simulink model "Connor"  (R2022b)
settings: Solver=VariableStepAuto  StartTime=0.0  StopTime=1  MaxStep=0.0001  RelTol=1e-3
values from neighbouring files (symbols this model uses):
  batteryTempCurve = (1 - batteryCoef *      (batteryTempX / maxBatteryTemp) .^ 2)    [red_crayon.m]
  batteryTempX = 0 : maxBatteryTemp / STEP_SIZE : maxBatteryTemp    [red_crayon.m]
  motorTempCurve = 150 -  (motorTempX - minMotorTemp) .^ 2 .* (150) / (maxMotorTemp - minMotorTemp)^2    [red_crayon.m]
  motorTempX = minMotorTemp : (maxMotorTemp-minMotorTemp) / STEP_SIZE : maxMotorTemp    [red_crayon.m]
undefined symbols (not defined in the file or in its folder): CENTER_STEER_ANGLE_MAX, deadband_angle, theta_left, theta_right, theta_sweep
libraries: dspstat3 x1
settings Model: Creator=Inver  LastModifiedBy=dagge
settings ModelReferenceCC: EnableRefExpFcnMdlSchedulingChecks=on

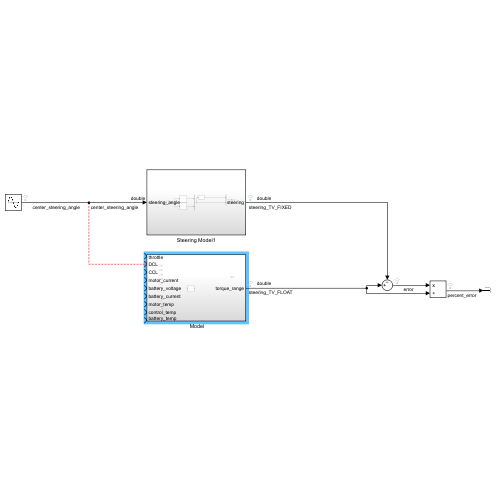
[thumbnail: Simulink's stored preview of the top-level diagram]
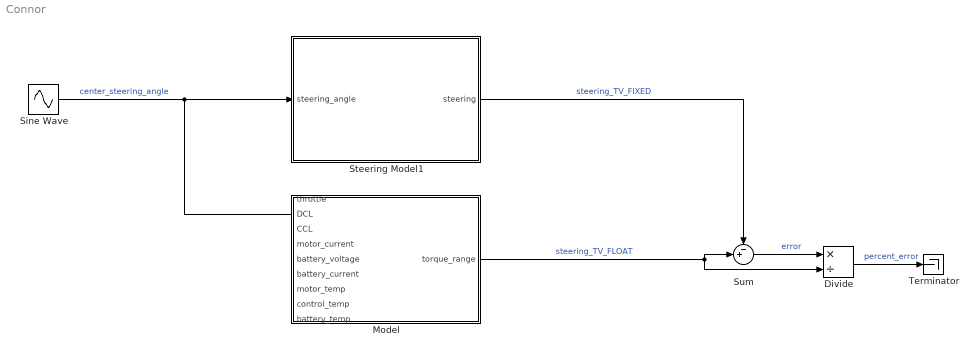
== system Connor ==
  " Model" : Subsystem
  Divide : Product  Inputs=*/
  Sine Wave : Sin  Amplitude=CENTER_STEER_ANGLE_MAX  Frequency=2*pi  SampleTime=0
  Steering Model1 : Subsystem
  Sum : Sum  Inputs=-+|
  Terminator : Terminator
  wires:
  Sum/1 -> Divide/1  "error"
  Divide/1 -> Terminator/1  "percent_error"
  " Model"/1(torque_range) -> Sum/2, Divide/2  "steering_TV_FLOAT"
  Sine Wave/1 -> Steering Model1/1(steering_angle)  "center_steering_angle"
  Steering Model1/1(steering) -> Sum/1  "steering_TV_FIXED"

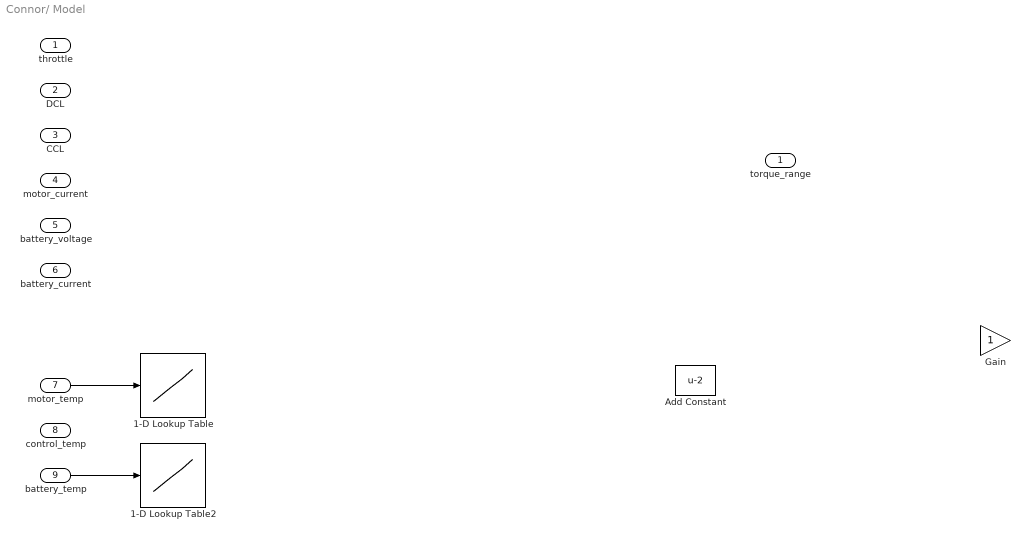
== system Connor/ Model ==
  throttle : Inport
  DCL : Inport  Port=2
  CCL : Inport  Port=3
  motor_current : Inport  Port=4
  battery_voltage : Inport  Port=5
  battery_current : Inport  Port=6
  motor_temp : Inport  Port=7
  control_temp : Inport  Port=8
  battery_temp : Inport  Port=9
  1-D Lookup Table : Lookup_n-D  NumberOfTableDimensions=1  BreakpointsForDimension1=motorTempX  Table=motorTempCurve  ExtrapMethod=Clip  UseLastTableValue=on  InternalRulePriority=Speed  RndMeth=Simplest
  1-D Lookup Table2 : Lookup_n-D  NumberOfTableDimensions=1  BreakpointsForDimension1=batteryTempX  Table=batteryTempCurve  ExtrapMethod=Clip  UseLastTableValue=on  InternalRulePriority=Speed  RndMeth=Simplest
  Add Constant : Bias  Bias=-2  SaturateOnIntegerOverflow=off
  Gain : Gain
  torque_range : Outport  OutDataTypeStr=double  LockScale=on
  wires:
  motor_temp/1 -> 1-D Lookup Table/1
  battery_temp/1 -> 1-D Lookup Table2/1

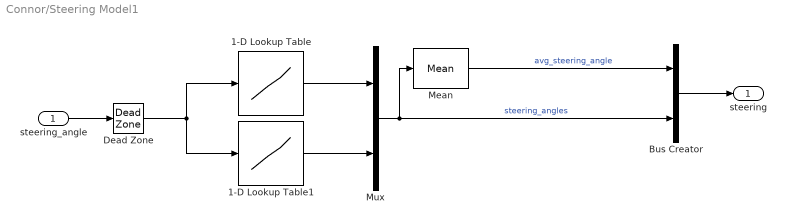
== system Connor/Steering Model1 ==
  steering_angle : Inport  OutMin=-130  OutMax=130  OutDataTypeStr=double  LockScale=on
  1-D Lookup Table : Lookup_n-D  NumberOfTableDimensions=1  BreakpointsForDimension1=theta_sweep  Table=theta_left  InterpMethod=Cubic spline  InternalRulePriority=Speed  RndMeth=Simplest
  1-D Lookup Table1 : Lookup_n-D  NumberOfTableDimensions=1  BreakpointsForDimension1=theta_sweep  Table=theta_right  InterpMethod=Cubic spline  InternalRulePriority=Speed  RndMeth=Simplest
  Bus Creator : BusCreator  Inputs=2
  Dead Zone : DeadZone  LowerValue=-deadband_angle  UpperValue=deadband_angle
  Mean : dspstat3/Mean  run=off  InputProcessing=Columns as channels (frame based)  reset_popup=None  directionMode=Each column  dimension=1  roiEnable=off  roiType=Rectangles  roiPortion=Entire ROI  roiOutput=Individual statistics for each ROI  roiFlag=off  roundingMode=Floor  overflowMode=off  outputDataTypeStr=Inherit: Same as accumulator  outputMin=[]  outputMax=[]  outputLastDataTypeStr=Inherit: Same as accumulator
  Mux : Mux  Inputs=2
  steering : Outport  OutDataTypeStr=double  LockScale=on
  wires:
  1-D Lookup Table/1 -> Mux/1
  Mean/1 -> Bus Creator/1  "avg_steering_angle"
  Mux/1 -> Bus Creator/2, Mean/1  "steering_angles"
  1-D Lookup Table1/1 -> Mux/2
  Bus Creator/1 -> steering/1
  steering_angle/1 -> Dead Zone/1
  Dead Zone/1 -> 1-D Lookup Table1/1, 1-D Lookup Table/1
